simulink model "planta10"  (Simulink 5.0)
settings: Solver=ode45  StartTime=0.0  StopTime=30  RelTol=1e-6
libraries: slident x1
settings Model: LastModifiedBy=Administrador

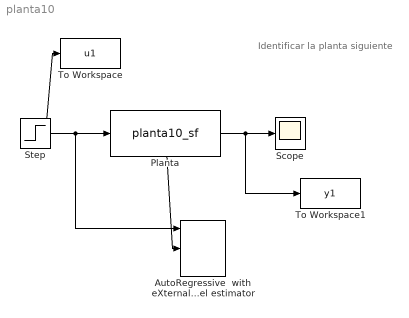
== system planta10 ==
  note: Identificar la planta siguiente
  AutoRegressive  with eXternal input model estimator : slident/AutoRegressive  with eXternal input model estimator  MaskParam1=256  MaskParam2=[8 9 0]  MaskParam3=64  MaskParam4=0.05
  Planta : S-Function  FunctionName=planta10_sf  SFunctionModules=""  mask{rtw_sf_name=planta10_sf, showVar=off}
      mask prompts: rtw_sf_name "Generated S-function name (model_sf):"; showVar "Show module list"
      mask help: Real-Time Workshop generated S-function.
      mask init:
      | displist = '';
      | if ~strcmp(get_param(gcb, 'FunctionName'), rtw_sf_name);
      |   set_param(gcb, 'FunctionName', rtw_sf_name);
      | end
      | if  showVar & exist('rtwsfunc') == 2
      |   tmplist = rtwsfunc(rtw_sf_name,gcb);
      |   tmplist = ['\nList of Modules:\n', tmplist];
      | elseif showVar
      |   tmplist = '\nList of Modules:\nRTW not licensed\n';
      | end
      | if showVar
      |   displist = tmplist;
      | end
      settings: CopyFcn=set_param(gcb,'linkstatus','none')
      mask Help: web(['file://',docroot,'/toolbox/rtw/rtwsfcn.html']);
      mask Display:
      | port_label('input',1,'u(t)');
      | port_label('output',1,'y(t)');
  Scope : Scope
  Step : Step  Time=0  SampleTime=0
  To Workspace : ToWorkspace  VariableName=u1  SampleTime=0.05  SaveFormat=Array
  To Workspace1 : ToWorkspace  VariableName=y1  SampleTime=0.05  SaveFormat=Array
  wires:
  Step/1 -> Planta/1, AutoRegressive  with eXternal input model estimator/1, To Workspace/1
  Planta/1 -> Scope/1, AutoRegressive  with eXternal input model estimator/2, To Workspace1/1
